simulink model "shifter_system_sim_new"  (R2018b)
settings: Solver=VariableStepAuto  StartTime=0.0  StopTime=10.0  RelTol=1e-3
values from neighbouring files (symbols this model uses):
  b = .05    (= 0.05)    [shifter_system_exec.m]
  J = .00082    (= 0.00082)    [shifter_system_exec.m]
  Ke = 2.47    [shifter_system_exec.m]
  Kt = 3.34    [shifter_system_exec.m]
  L = 1    [shifter_system_exec.m]
  R = 1.17    [shifter_system_exec.m]
libraries: simulink x2, dspstat3 x1
settings Model: Creator=michaelscirocco  LastModifiedBy=michaelscirocco

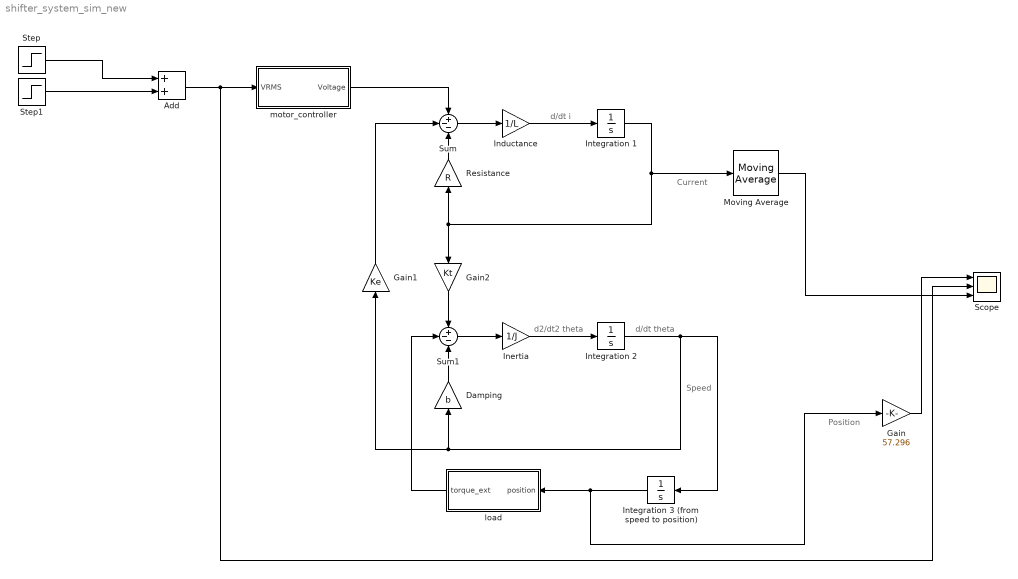
== system shifter_system_sim_new ==
  note: Position
  note: Speed
  note: Current
  note: d2/dt2 theta
  note: d/dt i
  note: d/dt theta
  Add : Sum
  Damping : Gain  Gain=b
  Gain : Gain  Gain=57.296
  Gain1 : Gain  Gain=Ke
  Gain2 : Gain  Gain=Kt
  Inductance : Gain  Gain=1/L
  Inertia : Gain  Gain=1/J
  "Integration 1 " : Integrator
  Integration 2 : Integrator
  Integration 3 (from speed to position) : Integrator
  Moving Average : dspstat3/Moving Average  Method=Sliding window  ForgettingFactorPort=off  SpecifyWindowLength=on  WindowLength=4  ForgettingFactor=0.9  SimulateUsing=Code generation
  Resistance : Gain  Gain=R
  Scope : Scope  NumInputPorts=3
  Step : Step  After=1.125  SampleTime=0
  Step1 : Step  Time=2  After=3.875  SampleTime=0
  Sum : Sum  Inputs=+--
  Sum1 : Sum  Inputs=+--
  load : Subsystem
  motor_controller : Subsystem
  wires:
  Add/1 -> Scope/2, motor_controller/1(VRMS)
  Step/1 -> Add/1
  Step1/1 -> Add/2
  motor_controller/1(Voltage) -> Sum/1
  Sum/1 -> Inductance/1
  Inductance/1 -> "Integration 1 "/1
  "Integration 1 "/1 -> Moving Average/1, Gain2/1, Resistance/1
  Resistance/1 -> Sum/3
  Gain2/1 -> Sum1/1
  Sum1/1 -> Inertia/1
  Inertia/1 -> Integration 2/1
  Integration 2/1 -> Gain1/1, Damping/1, Integration 3 (from speed to position)/1
  Gain1/1 -> Sum/2
  Damping/1 -> Sum1/3
  Integration 3 (from speed to position)/1 -> Gain/1, load/1(position)
  load/1(torque_ext) -> Sum1/2
  Gain/1 -> Scope/1
  Moving Average/1 -> Scope/3

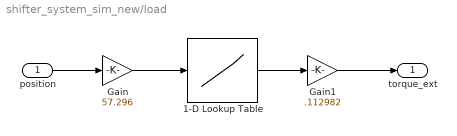
== system shifter_system_sim_new/load ==
  position : Inport
  1-D Lookup Table : Lookup_n-D  NumberOfTableDimensions=1  BreakpointsForDimension1=[0, 0.1, 58, 58.1]  Table=[0, 61, 76.25 , 100]  InternalRulePriority=Speed  RndMeth=Simplest  InputSameDT=on
  Gain : Gain  Gain=57.296
  Gain1 : Gain  Gain=.112982
  torque_ext : Outport
  wires:
  position/1 -> Gain/1
  1-D Lookup Table/1 -> Gain1/1
  Gain/1 -> 1-D Lookup Table/1
  Gain1/1 -> torque_ext/1

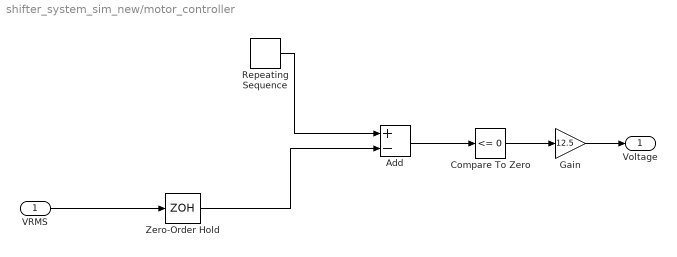
== system shifter_system_sim_new/motor_controller ==
  VRMS : Inport
  Add : Sum  Inputs=+-
  Compare To Zero : simulink/Logic and Bit Operations/Compare To Zero  relop=<=  OutDataTypeStr=boolean
  Gain : Gain  Gain=12.5
  Repeating Sequence : simulink/Sources/Repeating Sequence  rep_seq_t=[0 .01]  rep_seq_y=[0 5]
  Zero-Order Hold : ZeroOrderHold  SampleTime=.01
  Voltage : Outport
  wires:
  VRMS/1 -> Zero-Order Hold/1
  Zero-Order Hold/1 -> Add/2
  Repeating Sequence/1 -> Add/1
  Compare To Zero/1 -> Gain/1
  Add/1 -> Compare To Zero/1
  Gain/1 -> Voltage/1
